simulink model "llm_inferencing_control copy"  (R2025b)
settings: Solver=FixedStepDiscrete  StartTime=0.0  StopTime=30  FixedStep=perturbed.dt  RelTol=1e-3
undefined symbols (not defined in the file): controller, perturbed
settings Model: Creator=hvasudevan  LastModifiedBy=hvasudevan

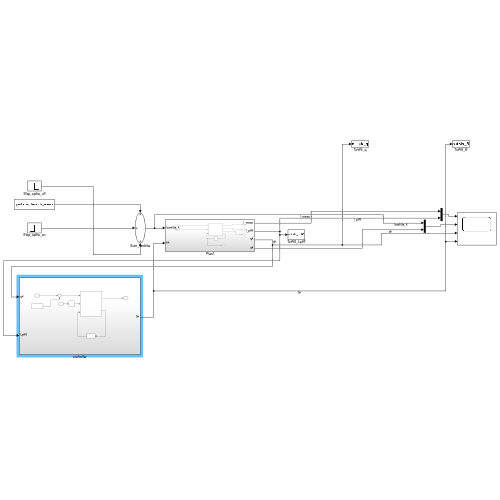
[thumbnail: Simulink's stored preview of the top-level diagram]
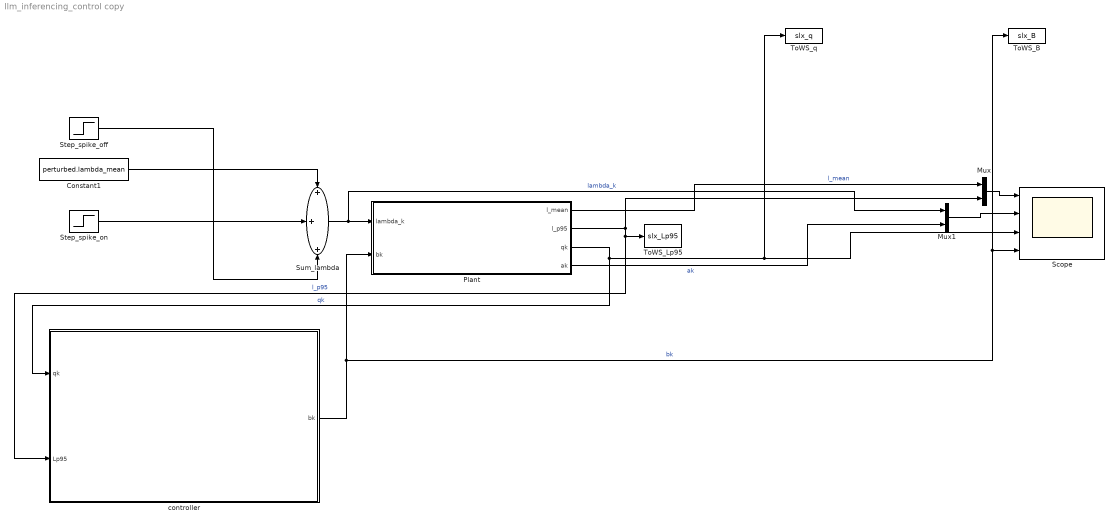
== system llm_inferencing_control copy ==
  Constant1 : Constant  Value=perturbed.lambda_mean  SampleTime=perturbed.dt
  Mux : Mux  Inputs=2
  Mux1 : Mux  Inputs=2
  Plant : Subsystem
  Scope : Scope  NumInputPorts=4
      settings: ActiveDisplayYMinimum=737.83102230791394  ActiveDisplayYMaximum=843.82042735729215
  Step_spike_off : Step  Time=15  After=-perturbed.lambda_mean  SampleTime=perturbed.dt
  Step_spike_on : Step  Time=5  After=perturbed.lambda_mean  SampleTime=perturbed.dt
  Sum_lambda : Sum  Inputs=+++
  ToWS_B : ToWorkspace  VariableName=slx_B  SampleTime=-1
  ToWS_Lp95 : ToWorkspace  VariableName=slx_Lp95  SampleTime=-1
  ToWS_q : ToWorkspace  VariableName=slx_q  SampleTime=-1
  controller : Subsystem
  wires:
  Step_spike_off/1 -> Sum_lambda/3
  Plant/3(qk) -> controller/1(qk), Scope/3, ToWS_q/1  "qk"
  Plant/2(l_p95) -> Mux/2, controller/2(Lp95), ToWS_Lp95/1  "l_p95"
  Plant/1(l_mean) -> Mux/1  "l_mean"
  Step_spike_on/1 -> Sum_lambda/2
  Constant1/1 -> Sum_lambda/1
  Sum_lambda/1 -> Mux1/1, Plant/1(lambda_k)  "lambda_k"
  Mux/1 -> Scope/1
  Mux1/1 -> Scope/2
  Plant/4(ak) -> Mux1/2  "ak"
  controller/1(bk) -> Plant/2(bk), Scope/4, ToWS_B/1  "bk"

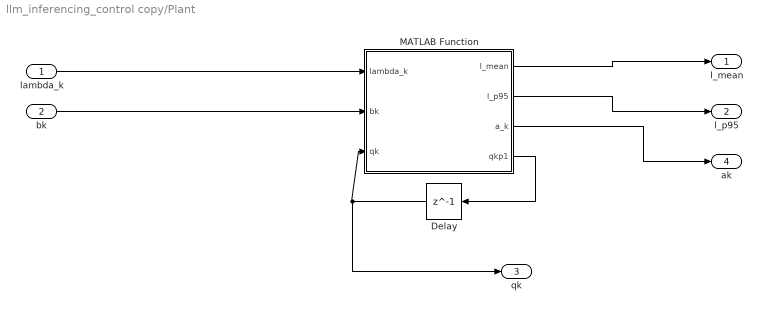
== system llm_inferencing_control copy/Plant ==
  lambda_k : Inport
  bk : Inport  Port=2
  Delay : Delay  DelayLength=1  InitialCondition=controller.q_eq  InputProcessing=Columns as channels (frame based)
  MATLAB Function : MATLAB Function  TreatAsAtomicUnit=on
  l_mean : Outport
  l_p95 : Outport  Port=2
  qk : Outport  Port=3
  ak : Outport  Port=4
  wires:
  MATLAB Function/2(l_p95) -> l_p95/1
  Delay/1 -> qk/1, MATLAB Function/3(qk)
  bk/1 -> MATLAB Function/2(bk)
  MATLAB Function/4(qkp1) -> Delay/1
  lambda_k/1 -> MATLAB Function/1(lambda_k)
  MATLAB Function/1(l_mean) -> l_mean/1
  MATLAB Function/3(a_k) -> ak/1

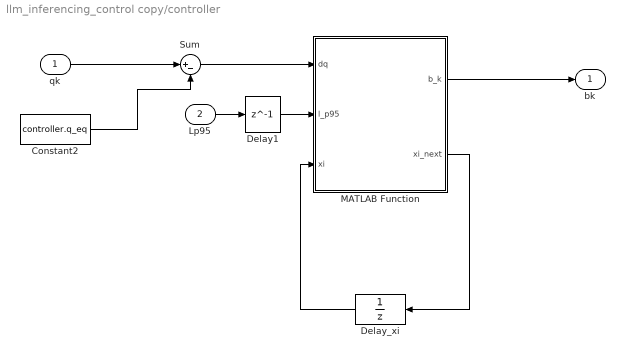
== system llm_inferencing_control copy/controller ==
  qk : Inport
  Lp95 : Inport  Port=2
  Constant2 : Constant  Value=controller.q_eq  SampleTime=perturbed.dt
  Delay1 : Delay  DelayLength=1  InitialCondition=controller.l_target  InputProcessing=Columns as channels (frame based)
  Delay_xi : UnitDelay  SampleTime=0.1  HasFrameUpgradeWarning=on
  MATLAB Function : MATLAB Function  TreatAsAtomicUnit=on
  Sum : Sum  Inputs=|+-
  bk : Outport
  wires:
  Sum/1 -> MATLAB Function/1(dq)
  Lp95/1 -> Delay1/1
  Delay_xi/1 -> MATLAB Function/3(xi)
  MATLAB Function/1(b_k) -> bk/1
  MATLAB Function/2(xi_next) -> Delay_xi/1
  Constant2/1 -> Sum/2
  qk/1 -> Sum/1
  Delay1/1 -> MATLAB Function/2(l_p95)

== matlab function llm_inferencing_control copy/controller/MATLAB Function ==
  data: dq input; b_k output; l_p95 input; xi input; xi_next output; controller parameter
function [b_k, xi_next] = direct_ctrl(dq, l_p95, xi, controller)
%DIRECT_CTRL  Direct b->l_p95 integral state-feedback controller — chapter 2.
%
%  inputs
%    dq          deviation of queue from equilibrium: dq = q[k] - q_eq
%    l_p95       measured rolling p95 latency [ms]
%    xi          integrator state xi[k] (integral of latency error)
%    controller  parameter struct from design_controller.m
%
%  outputs
%    b_k         batch size command b[k]  (clamped to [b_min, b_max])
%    xi_next     updated integrator state xi[k+1]
%
% =========================================================================
% augmented state and control law
% =========================================================================
%
%  state:   x[k] = [dq[k] ; xi[k]]
%
%  control law (state feedback):
%    db[k] = -k_q * dq[k]  -  k_i * xi[k]
%    b[k]  = b_eq + db[k]      clamped to [b_min, b_max]
%
% =========================================================================
% normal integrator
% =========================================================================
%
%  unlike the model-based update which used the linearised output equation
%  to propagate latency error into xi, here we integrate the actual
%  measured latency error directly:
%
%    e[k]    = l_target - l_p95[k]      (positive when latency too low,
%                                         negative when latency too high)
%    xi[k+1] = xi[k] + e[k]
%
%  this is the standard integrator used in classical pi/integral
%  state-feedback control.  it has no dependence on the plant model
%  parameters beta or c1 — the only signal it uses is the measured
%  output l_p95 and the reference l_target.
%
%  the tradeoff vs model-based: this integrator accumulates the rolling
%  buffer lag (~6s window) directly into xi, so it is slower to respond.
%  but it is robust to model mismatch and does not require knowledge of
%  c1 or beta to stay bounded.
%
%  conditional anti-windup: freeze xi when b is saturated, to prevent
%  the integrator winding in a direction the actuator cannot follow.
%
% =========================================================================

% -- unpack controller struct ----------------------------------------------
k_q      = controller.k_q;       % state feedback gain on dq
k_i      = controller.k_i;       % integral gain on xi
b_eq     = controller.b_eq;      % equilibrium batch size [req/tick]
b_min    = controller.b_min;     % actuator lower bound
b_max    = controller.b_max;     % actuator upper bound
xi_max   = controller.xi_max;    % anti-windup ceiling on xi
xi_min   = controller.xi_min;    % anti-windup floor on xi
l_target = controller.l_target;  % latency reference [ms]
q_max    = controller.q_max;     % dq saturation bound

% -- saturate dq -----------------------------------------------------------
%
%  clamp dq to [-q_max, q_max] to keep the proportional term within
%  the region where the jacobian linearisation is valid.
dq_sat = min(max(dq, -q_max), q_max);

% -- control law -----------------------------------------------------------
%
%  db[k] = -k_q * dq[k] - k_i * xi[k]
%  b[k]  = b_eq + db[k]   clamped to [b_min, b_max]
db      = -k_q * dq_sat - k_i * xi;
b_unsat = b_eq + db;
b_k     = min(b_max, max(b_min, b_unsat));

% -- latency error for integrator ------------------------------------------
%
%  e[k] = l_target - l_p95[k]
%  positive e: latency below target, xi winds positive, integral term
%              reduces b (since k_i > 0 from lqr => -k_i*xi < 0 => db < 0)
%  negative e: latency above target, xi winds negative, integral term
%              increases b to drain queue and lower latency
e_L = l_target - l_p95;

% -- integrator update with conditional anti-windup ------------------------
%
%  unsaturated: xi[k+1] = xi[k] + e[k]    (clipped to [xi_min, xi_max])
%  saturated:   xi[k+1] = xi[k]           (freeze — no further wind-up)
if b_unsat == b_k
    xi_next = min(xi_max, max(xi_min, xi + e_L));
else
    xi_next = xi;
end

end

== matlab function llm_inferencing_control copy/Plant/MATLAB Function ==
  data: lambda_k input; bk input; l_mean output; qk input; l_p95 output; a_k output; qkp1 output; perturbed parameter
function [l_mean, l_p95, a_k, qkp1] = fcn(lambda_k, bk, qk, perturbed)
%% STATISTICAL PLANT - Chapter 2
%% Replaces deterministic arrivals and closed-form p95 with:
%%   - True Poisson arrivals: a[k] ~ Poisson(lambda_k)
%%   - Per-tick latency sample with additive noise
%%   - Empirical rolling p95 over a 60-sample window
%%
%% Everything else (queue equation, latency formula, parameters)
%% is identical to Chapter 1.

persistent L_buf buf_idx buf_full
N = 60;
if isempty(L_buf)
    %% Warm-start buffer at target so outer loop sees zero error at t=0.
    %% Without this the cold buffer reads L_p95~0 and winds the integrator.
    L_buf    = perturbed.L_p95_target * ones(1, N);
    buf_idx  = 0;
    buf_full = true;
end

alpha = perturbed.alpha;
gam   = perturbed.gamma;
beta  = perturbed.beta;
delta = perturbed.delta;

%% True Poisson arrivals (not Gaussian approx — avoids fat-tail spikes)
a_k = poissrnd(max(0, lambda_k));

%% Queue state equation — identical to Chapter 1
qkp1 = max(0, qk + a_k - bk);

%% Latency sample this tick
bk_safe = max(1, bk);
l_det   = alpha*bk + gam*bk^2 + beta*qk;
l_samp  = l_det + (delta / sqrt(bk_safe)) * randn();

%% Update circular buffer
buf_idx = mod(buf_idx, N) + 1;
L_buf(buf_idx) = l_samp;

%% Rolling statistics
if buf_full
    data = L_buf;
else
    data = L_buf(1 : buf_idx);
end

l_mean = mean(data);
sorted = sort(data);
idx95  = max(1, ceil(0.95 * length(sorted)));
l_p95  = sorted(idx95);

end
